simulink model "mobile_robot_model"  (R2020a)
settings: Solver=ode4  StartTime=0.0  StopTime=10.0  FixedStep=0.1  RelTol=1e-3
values from neighbouring files (symbols this model uses):
  L = 1    [mobile_robots.m]
undefined symbols (not defined in the file or in its folder): sigbuilder_block
libraries: simulink x1
settings Model: Creator=krzysztof  LastModifiedBy=krzysztof

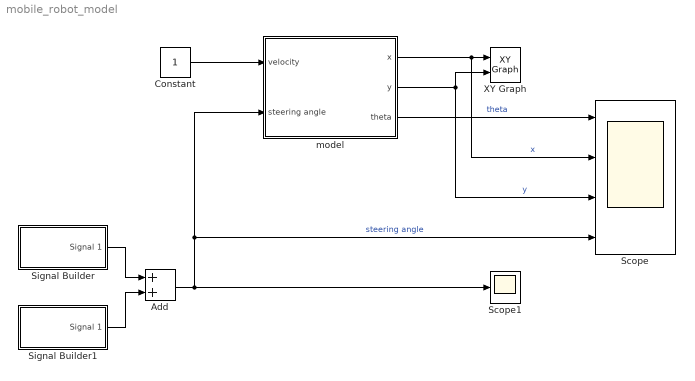
== system mobile_robot_model ==
  Add : Sum
  Constant : Constant
  Scope : Scope  NumInputPorts=4
  Scope1 : Scope
  Signal Builder : Subsystem  Tag=STV Subsys  LoadFcn=sigbuilder_block('load');  StartFcn=sigbuilder_block('start');  StopFcn=sigbuilder_block('stop');  ClipboardFcn=sigbuilder_block('clipboard');  mask(Sigbuilder block){tuvar=[0:10]}
      mask help: Simulink:masks:SigbuilderBlock_MD
      mask init:
      | if ~strcmp(get_param(bdroot(gcbh),'SimulationStatus'),'stopped') tuvar = sigbuilder_block('maskInit'); end
      settings: CopyFcn=sigbuilder_block('copy');  DeleteFcn=sigbuilder_block('delete');  ModelCloseFcn=sigbuilder_block('modelClose');  PreSaveFcn=sigbuilder_block('preSave');  PauseFcn=sigbuilder_block('pause');  ContinueFcn=sigbuilder_block('continue');  NameChangeFcn=sigbuilder_block('namechange');  OpenFcn=sigbuilder_block('open',[437.6 199.2 550.4 400 ]);  CloseFcn=sigbuilder_block('close');
      mask Display: plot(0, 0, 100, 100,[2, 2, 32, 32, 2], [68, 8, 8, 68, 68],[32, 2], [38, 38], [32, 19, 2],[53, 60, 44], [32, 17, 17, 2],[16, 16, 31, 31]);txt = getActiveGroup(gcbh);text(2, 100, txt,'verticalAlignment', 'top');
  Signal Builder1 : Subsystem  Tag=STV Subsys  LoadFcn=sigbuilder_block('load');  StartFcn=sigbuilder_block('start');  StopFcn=sigbuilder_block('stop');  ClipboardFcn=sigbuilder_block('clipboard');  mask(Sigbuilder block){tuvar=[0:10]}
      mask help: Simulink:masks:SigbuilderBlock_MD
      mask init:
      | if ~strcmp(get_param(bdroot(gcbh),'SimulationStatus'),'stopped') tuvar = sigbuilder_block('maskInit'); end
      settings: CopyFcn=sigbuilder_block('copy');  DeleteFcn=sigbuilder_block('delete');  ModelCloseFcn=sigbuilder_block('modelClose');  PreSaveFcn=sigbuilder_block('preSave');  PauseFcn=sigbuilder_block('pause');  ContinueFcn=sigbuilder_block('continue');  NameChangeFcn=sigbuilder_block('namechange');  OpenFcn=sigbuilder_block('open',[437.6 199.2 550.4 400 ]);  CloseFcn=sigbuilder_block('close');
      mask Display: plot(0, 0, 100, 100,[2, 2, 32, 32, 2], [68, 8, 8, 68, 68],[32, 2], [38, 38], [32, 19, 2],[53, 60, 44], [32, 17, 17, 2],[16, 16, 31, 31]);txt = getActiveGroup(gcbh);text(2, 100, txt,'verticalAlignment', 'top');
  XY Graph : simulink/Sinks/XY Graph  xmin=0  xmax=10  ymin=0  ymax=10  st=-1
  model : Subsystem
  wires:
  Constant/1 -> model/1(velocity)
  Signal Builder/1(Signal 1) -> Add/1
  Signal Builder1/1(Signal 1) -> Add/2
  model/3(theta) -> Scope/1  "theta"
  model/1(x) -> Scope/2, XY Graph/1  "x"
  model/2(y) -> XY Graph/2, Scope/3  "y"
  Add/1 -> model/2(steering angle), Scope/4, Scope1/1  "steering angle"

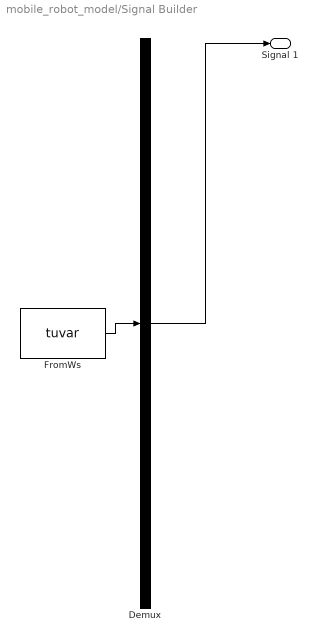
== system mobile_robot_model/Signal Builder ==
  Demux : Demux  Tag=STV Demux  Outputs=1
      settings: DisplayOption=none
  FromWs : FromWorkspace  Tag=STV FromWs  VariableName=tuvar
      SigBuilderData=|
      | common.afterFinalStr = 'Extrapolate'
      | common.sampleTime = 0
      | dataSet.timeRange = [0 10]
      | dataSet.name = 'Group 1'
      | sbobj.Groups.Name = 'Group 1'
      | sbobj.Groups.Signals.Name = 'Signal 1'
      | sbobj.Groups.Signals.XData = [0 3 3 4 4 10]
      | sbobj.Groups.Signals.YData = [0 0 0.5 0.5 0 0]
  Signal 1 : Outport  Tag=STV Outport
  wires:
  Demux/1 -> Signal 1/1
  FromWs/1 -> Demux/1

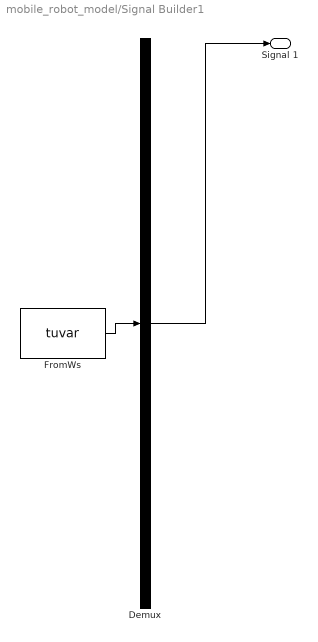
== system mobile_robot_model/Signal Builder1 ==
  Demux : Demux  Tag=STV Demux  Outputs=1
      settings: DisplayOption=none
  FromWs : FromWorkspace  Tag=STV FromWs  VariableName=tuvar
      SigBuilderData=|
      | common.afterFinalStr = 'Extrapolate'
      | common.sampleTime = 0
      | dataSet.timeRange = [0 10]
      | dataSet.name = 'Group 1'
      | sbobj.Groups.Name = 'Group 1'
      | sbobj.Groups.Signals.Name = 'Signal 1'
      | sbobj.Groups.Signals.XData = [0 5 5 6 6 10]
      | sbobj.Groups.Signals.YData = [0 0 -0.5 -0.5 0 0]
  Signal 1 : Outport  Tag=STV Outport
  wires:
  Demux/1 -> Signal 1/1
  FromWs/1 -> Demux/1

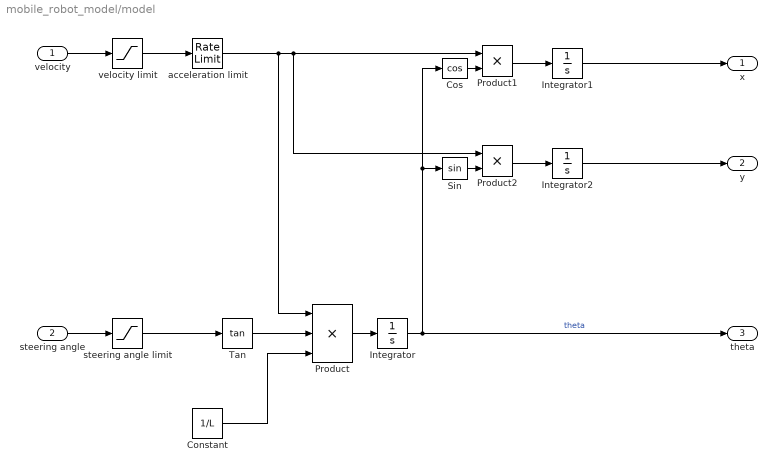
== system mobile_robot_model/model ==
  velocity : Inport
  steering angle : Inport  Port=2
  Constant : Constant  Value=1/L
  Cos : Trigonometry  Operator=cos  OutputSignalType=real
  Integrator : Integrator
  Integrator1 : Integrator
  Integrator2 : Integrator
  Product : Product  Inputs=3
  Product1 : Product
  Product2 : Product
  Sin : Trigonometry  OutputSignalType=real
  Tan : Trigonometry  Operator=tan
  acceleration limit : RateLimiter  SampleTimeMode=inherited
  steering angle limit : Saturate  UpperLimit=1  LowerLimit=-1  LinearizeAsGain=off
  velocity limit : Saturate  UpperLimit=2  LowerLimit=-2
  x : Outport
  y : Outport  Port=2
  theta : Outport  Port=3
  wires:
  Product1/1 -> Integrator1/1
  Integrator2/1 -> y/1
  Product2/1 -> Integrator2/1
  Integrator/1 -> theta/1, Cos/1, Sin/1  "theta"
  Integrator1/1 -> x/1
  Cos/1 -> Product1/2
  Tan/1 -> Product/2
  Constant/1 -> Product/3
  steering angle limit/1 -> Tan/1
  acceleration limit/1 -> Product/1, Product2/1, Product1/1
  Sin/1 -> Product2/2
  Product/1 -> Integrator/1
  steering angle/1 -> steering angle limit/1
  velocity limit/1 -> acceleration limit/1
  velocity/1 -> velocity limit/1
